simulink model "TST_FlSys_FlConsTot"  (R2016b)
settings: Solver=FixedStepDiscrete  StartTime=0.0  StopTime=simTime  FixedStep=sampleTime  RelTol=1e-3
values from neighbouring files (symbols this model uses):
  testCase = 1    [initTST_FlSys_FlConsTot_001.m]
libraries: simulink x4, UnitTest_Lib x2
settings Model: Creator=zhengjinyan  LastModifiedBy=zhengjinyan
settings DebuggingCC: SignalRangeChecking=error

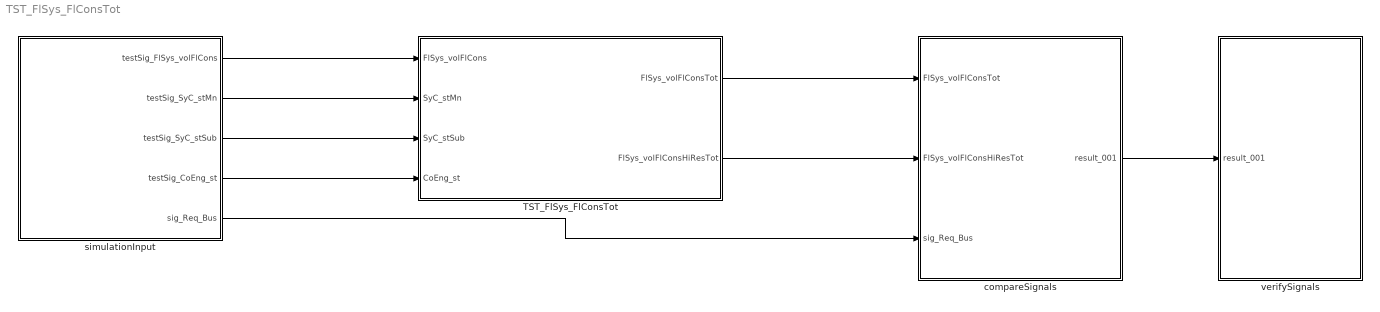
== system TST_FlSys_FlConsTot ==
  TST_FlSys_FlConsTot : Subsystem
  compareSignals : Subsystem
  simulationInput : Subsystem
  verifySignals : Subsystem
  wires:
  simulationInput/1(testSig_FlSys_volFlCons) -> TST_FlSys_FlConsTot/1(FlSys_volFlCons)
  simulationInput/2(testSig_SyC_stMn) -> TST_FlSys_FlConsTot/2(SyC_stMn)
  simulationInput/3(testSig_SyC_stSub) -> TST_FlSys_FlConsTot/3(SyC_stSub)
  simulationInput/4(testSig_CoEng_st) -> TST_FlSys_FlConsTot/4(CoEng_st)
  TST_FlSys_FlConsTot/1(FlSys_volFlConsTot) -> compareSignals/1(FlSys_volFlConsTot)
  TST_FlSys_FlConsTot/2(FlSys_volFlConsHiResTot) -> compareSignals/2(FlSys_volFlConsHiResTot)
  simulationInput/5(sig_Req_Bus) -> compareSignals/3(sig_Req_Bus)
  compareSignals/1(result_001) -> verifySignals/1(result_001)

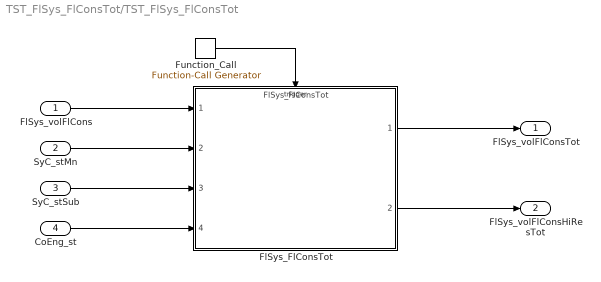
== system TST_FlSys_FlConsTot/TST_FlSys_FlConsTot ==
  FlSys_volFlCons : Inport
  SyC_stMn : Inport  Port=2
  SyC_stSub : Inport  Port=3
  CoEng_st : Inport  Port=4
  FlSys_FlConsTot : ModelReference  ModelNameDialog=FlSys_FlConsTot  SimulationMode=Normal  ModelReferenceVersion=1.14  TriggerPortName=function  TriggerPortTriggerType=function-call  TriggerPortStatesWhenEnabling=held
  Function_Call : simulink/Ports & Subsystems/Function-Call Generator  sample_time=sampleTime  numberOfIterations=1
  FlSys_volFlConsTot : Outport
  FlSys_volFlConsHiResTot : Outport  Port=2
  wires:
  Function_Call/1 -> FlSys_FlConsTot/Trigger
  FlSys_volFlCons/1 -> FlSys_FlConsTot/1
  SyC_stMn/1 -> FlSys_FlConsTot/2
  SyC_stSub/1 -> FlSys_FlConsTot/3
  CoEng_st/1 -> FlSys_FlConsTot/4
  FlSys_FlConsTot/1 -> FlSys_volFlConsTot/1
  FlSys_FlConsTot/2 -> FlSys_volFlConsHiResTot/1

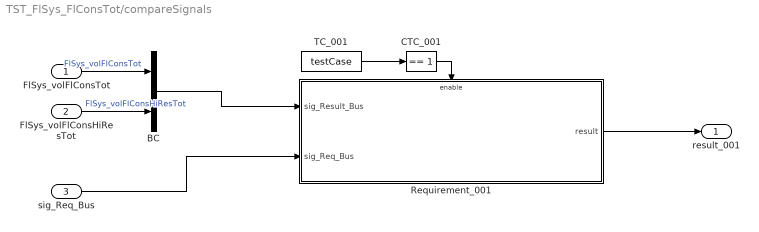
== system TST_FlSys_FlConsTot/compareSignals ==
  FlSys_volFlConsTot : Inport
  FlSys_volFlConsHiResTot : Inport  Port=2
  sig_Req_Bus : Inport  Port=3
  BC : BusCreator  Inputs=2
  CTC_001 : simulink/Logic and Bit Operations/Compare To Constant  relop===  const=1  OutDataTypeStr=boolean
  Requirement_001 : Subsystem
  TC_001 : Constant  Value=testCase
  result_001 : Outport
  wires:
  FlSys_volFlConsTot/1 -> BC/1  "FlSys_volFlConsTot"
  FlSys_volFlConsHiResTot/1 -> BC/2  "FlSys_volFlConsHiResTot"
  TC_001/1 -> CTC_001/1
  CTC_001/1 -> Requirement_001/Enable
  sig_Req_Bus/1 -> Requirement_001/2(sig_Req_Bus)
  BC/1 -> Requirement_001/1(sig_Result_Bus)
  Requirement_001/1(result) -> result_001/1

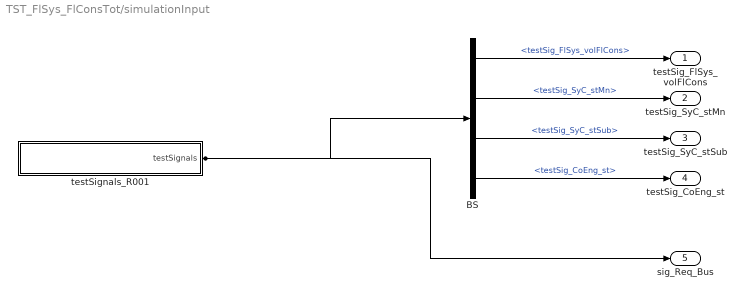
== system TST_FlSys_FlConsTot/simulationInput ==
  BS : BusSelector  OutputSignals=testSig_FlSys_volFlCons,testSig_SyC_stMn,testSig_SyC_stSub,testSig_CoEng_st
  testSignals_R001 : Subsystem
  testSig_FlSys_volFlCons : Outport
  testSig_SyC_stMn : Outport  Port=2
  testSig_SyC_stSub : Outport  Port=3
  testSig_CoEng_st : Outport  Port=4
  sig_Req_Bus : Outport  Port=5
  wires:
  BS/1 -> testSig_FlSys_volFlCons/1  "<testSig_FlSys_volFlCons>"
  BS/2 -> testSig_SyC_stMn/1  "<testSig_SyC_stMn>"
  BS/3 -> testSig_SyC_stSub/1  "<testSig_SyC_stSub>"
  BS/4 -> testSig_CoEng_st/1  "<testSig_CoEng_st>"
  testSignals_R001/1(testSignals) -> BS/1, sig_Req_Bus/1

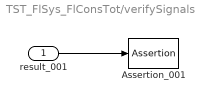
== system TST_FlSys_FlConsTot/verifySignals ==
  result_001 : Inport
  Assertion_001 : Assertion  Enabled=off
  wires:
  result_001/1 -> Assertion_001/1

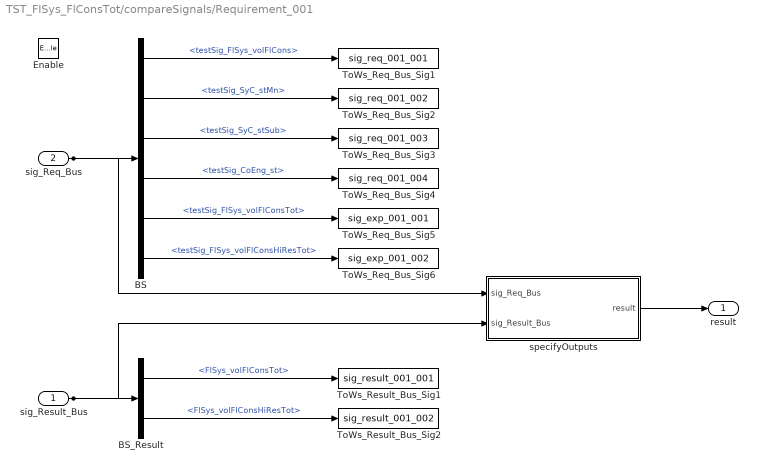
== system TST_FlSys_FlConsTot/compareSignals/Requirement_001 ==
  sig_Result_Bus : Inport
  sig_Req_Bus : Inport  Port=2
  Enable : EnablePort
  BS : BusSelector  OutputSignals=testSig_FlSys_volFlCons,testSig_SyC_stMn,testSig_SyC_stSub,testSig_CoEng_st,testSig_FlSys_volFlConsTot,testSig_FlSys_volFlConsHiResTot
  BS_Result : BusSelector  OutputSignals=FlSys_volFlConsTot,FlSys_volFlConsHiResTot
  ToWs_Req_Bus_Sig1 : ToWorkspace  VariableName=sig_req_001_001  SaveFormat=Structure With Time
  ToWs_Req_Bus_Sig2 : ToWorkspace  VariableName=sig_req_001_002  SaveFormat=Structure With Time
  ToWs_Req_Bus_Sig3 : ToWorkspace  VariableName=sig_req_001_003  SaveFormat=Structure With Time
  ToWs_Req_Bus_Sig4 : ToWorkspace  VariableName=sig_req_001_004  SaveFormat=Structure With Time
  ToWs_Req_Bus_Sig5 : ToWorkspace  VariableName=sig_exp_001_001  SaveFormat=Structure With Time
  ToWs_Req_Bus_Sig6 : ToWorkspace  VariableName=sig_exp_001_002  SaveFormat=Structure With Time
  ToWs_Result_Bus_Sig1 : ToWorkspace  VariableName=sig_result_001_001  SaveFormat=Structure With Time
  ToWs_Result_Bus_Sig2 : ToWorkspace  VariableName=sig_result_001_002  SaveFormat=Structure With Time
  specifyOutputs : Subsystem
  result : Outport
  wires:
  sig_Req_Bus/1 -> BS/1, specifyOutputs/1(sig_Req_Bus)
  BS/1 -> ToWs_Req_Bus_Sig1/1  "<testSig_FlSys_volFlCons>"
  BS/2 -> ToWs_Req_Bus_Sig2/1  "<testSig_SyC_stMn>"
  BS/3 -> ToWs_Req_Bus_Sig3/1  "<testSig_SyC_stSub>"
  BS/4 -> ToWs_Req_Bus_Sig4/1  "<testSig_CoEng_st>"
  BS/5 -> ToWs_Req_Bus_Sig5/1  "<testSig_FlSys_volFlConsTot>"
  BS/6 -> ToWs_Req_Bus_Sig6/1  "<testSig_FlSys_volFlConsHiResTot>"
  sig_Result_Bus/1 -> BS_Result/1, specifyOutputs/2(sig_Result_Bus)
  BS_Result/1 -> ToWs_Result_Bus_Sig1/1  "<FlSys_volFlConsTot>"
  BS_Result/2 -> ToWs_Result_Bus_Sig2/1  "<FlSys_volFlConsHiResTot>"
  specifyOutputs/1(result) -> result/1

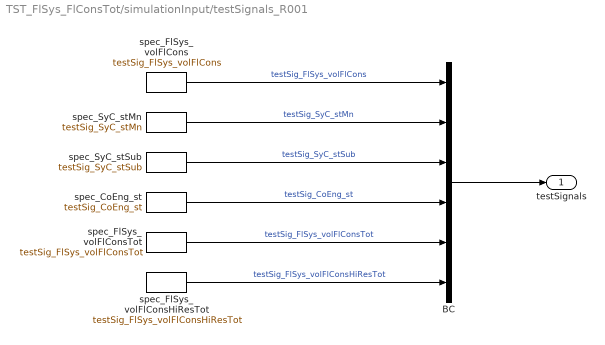
== system TST_FlSys_FlConsTot/simulationInput/testSignals_R001 ==
  BC : BusCreator  Inputs=6
  spec_CoEng_st : FromWorkspace  VariableName=testSig_CoEng_st  Interpolate=off  OutputAfterFinalValue=Holding final value
  spec_FlSys_volFlCons : FromWorkspace  VariableName=testSig_FlSys_volFlCons  Interpolate=off  OutputAfterFinalValue=Holding final value
  spec_FlSys_volFlConsHiResTot : FromWorkspace  VariableName=testSig_FlSys_volFlConsHiResTot  Interpolate=off  OutputAfterFinalValue=Holding final value
  spec_FlSys_volFlConsTot : FromWorkspace  VariableName=testSig_FlSys_volFlConsTot  Interpolate=off  OutputAfterFinalValue=Holding final value
  spec_SyC_stMn : FromWorkspace  VariableName=testSig_SyC_stMn  Interpolate=off  OutputAfterFinalValue=Holding final value
  spec_SyC_stSub : FromWorkspace  VariableName=testSig_SyC_stSub  Interpolate=off  OutputAfterFinalValue=Holding final value
  testSignals : Outport
  wires:
  BC/1 -> testSignals/1
  spec_FlSys_volFlCons/1 -> BC/1  "testSig_FlSys_volFlCons"
  spec_SyC_stMn/1 -> BC/2  "testSig_SyC_stMn"
  spec_SyC_stSub/1 -> BC/3  "testSig_SyC_stSub"
  spec_CoEng_st/1 -> BC/4  "testSig_CoEng_st"
  spec_FlSys_volFlConsTot/1 -> BC/5  "testSig_FlSys_volFlConsTot"
  spec_FlSys_volFlConsHiResTot/1 -> BC/6  "testSig_FlSys_volFlConsHiResTot"

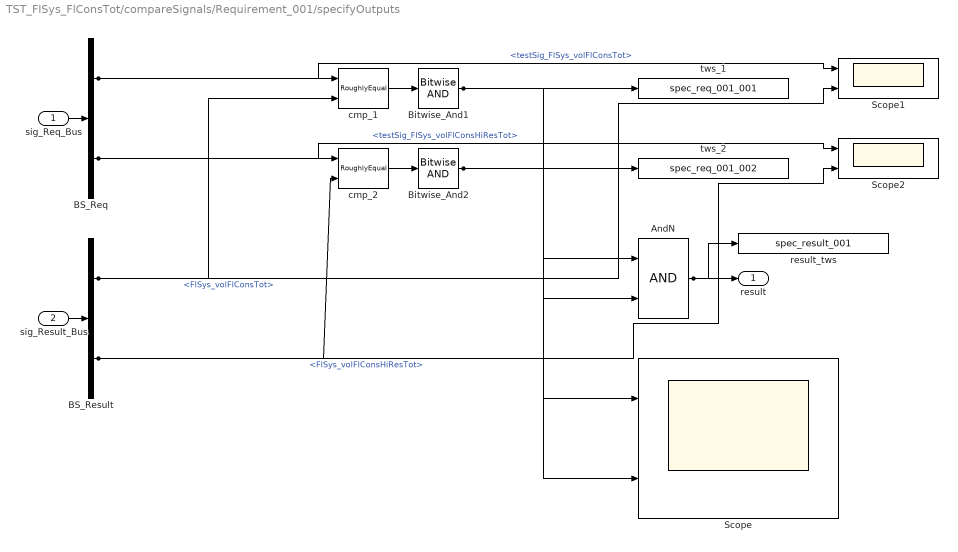
== system TST_FlSys_FlConsTot/compareSignals/Requirement_001/specifyOutputs ==
  sig_Req_Bus : Inport
  sig_Result_Bus : Inport  Port=2
  AndN : Logic
  BS_Req : BusSelector  OutputSignals=testSig_FlSys_volFlConsTot,testSig_FlSys_volFlConsHiResTot
  BS_Result : BusSelector  OutputSignals=FlSys_volFlConsTot,FlSys_volFlConsHiResTot
  Bitwise_And1 : simulink/Logic and Bit Operations/Bitwise Operator  logicop=AND  UseBitMask=off  BitMask=bin2dec('11011001')  BitMaskRealWorld=Stored Integer
  Bitwise_And2 : simulink/Logic and Bit Operations/Bitwise Operator  logicop=AND  UseBitMask=off  BitMask=bin2dec('11011001')  BitMaskRealWorld=Stored Integer
  Scope : Scope  NumInputPorts=2
  Scope1 : Scope  NumInputPorts=2
  Scope2 : Scope  NumInputPorts=2
  cmp_1 : UnitTest_Lib/RoughlyEqual  slope=0.1
  cmp_2 : UnitTest_Lib/RoughlyEqual  slope=0.1
  result_tws : ToWorkspace  VariableName=spec_result_001
  tws_1 : ToWorkspace  VariableName=spec_req_001_001
  tws_2 : ToWorkspace  VariableName=spec_req_001_002
  result : Outport
  wires:
  sig_Req_Bus/1 -> BS_Req/1
  sig_Result_Bus/1 -> BS_Result/1
  AndN/1 -> result/1, result_tws/1
  BS_Req/1 -> cmp_1/1, Scope1/1  "<testSig_FlSys_volFlConsTot>"
  BS_Result/1 -> cmp_1/2, Scope1/2  "<FlSys_volFlConsTot>"
  cmp_1/1 -> Bitwise_And1/1
  Bitwise_And1/1 -> tws_1/1, AndN/1, Scope/1
  BS_Req/2 -> cmp_2/1, Scope2/1  "<testSig_FlSys_volFlConsHiResTot>"
  BS_Result/2 -> cmp_2/2, Scope2/2  "<FlSys_volFlConsHiResTot>"
  cmp_2/1 -> Bitwise_And2/1
  Bitwise_And2/1 -> tws_2/1, AndN/2, Scope/2
